simulink model "pendubotSim"  (R2016a)
settings: Solver=VariableStepAuto  StartTime=0.0  StopTime=10.0  RelTol=1e-3
InitFcn:
  | initFcn
values from neighbouring files (symbols this model uses):
  g = 9.81    [getParams.m]    (also in sFunModell.m = block.DialogPrm(1).Data)
  l1 = 0.2    [getParams.m]    (also in sFunModell.m = block.DialogPrm(4).Data)
  l2 = 0.2    [getParams.m]    (also in sFunModell.m = block.DialogPrm(5).Data)
  m1 = 0.3    [getParams.m]    (also in sFunModell.m = block.DialogPrm(2).Data)
  m2 = 0.3    [getParams.m]    (also in sFunModell.m = block.DialogPrm(3).Data)
  RP1 = 1e-2    (= 0.01)    [getParams.m]    (also in sFunModell.m = block.DialogPrm(6).Data)
  RP2 = 1e-3    (= 0.001)    [getParams.m]    (also in sFunModell.m = block.DialogPrm(7).Data)
settings Model: Creator=bened  LastModifiedBy=bened
settings GRTTargetCC: GeneratePreprocessorConditionals=Use local settings

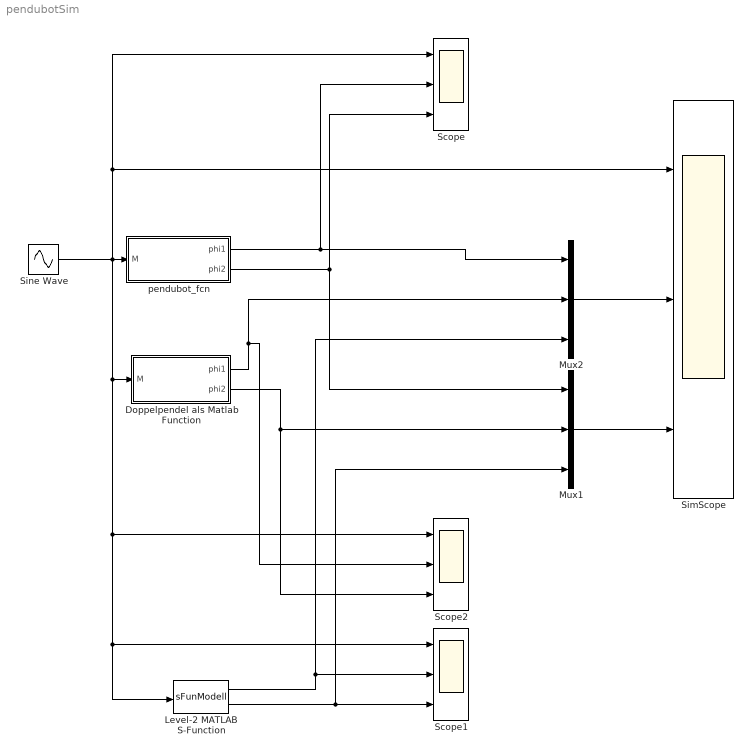
== system pendubotSim ==
  Doppelpendel als Matlab Function : Subsystem
  Level-2 MATLAB S-Function : M-S-Function  FunctionName=sFunModell  Parameters=g, m1, m2, l1, l2, RP1, RP2
  Mux1 : Mux  Inputs=3
  Mux2 : Mux  Inputs=3
  Scope : Scope  NumInputPorts=3
  Scope1 : Scope  NumInputPorts=3
  Scope2 : Scope  NumInputPorts=3
  "SimScope " : Scope  NumInputPorts=3
  Sine Wave : Sin  Amplitude=.1  SampleTime=0
  pendubot_fcn : Subsystem
  wires:
  pendubot_fcn/1(phi1) -> Mux2/1, Scope/2
  pendubot_fcn/2(phi2) -> Mux1/1, Scope/3
  Level-2 MATLAB S-Function/1 -> Mux2/3, Scope1/2
  Level-2 MATLAB S-Function/2 -> Scope1/3, Mux1/3
  Mux2/1 -> "SimScope "/2
  Mux1/1 -> "SimScope "/3
  Doppelpendel als Matlab Function/1(phi1) -> Scope2/2, Mux2/2
  Doppelpendel als Matlab Function/2(phi2) -> Scope2/3, Mux1/2
  Sine Wave/1 -> Doppelpendel als Matlab Function/1(M), Scope2/1, Level-2 MATLAB S-Function/1, Scope1/1, "SimScope "/1, Scope/1, pendubot_fcn/1(M)

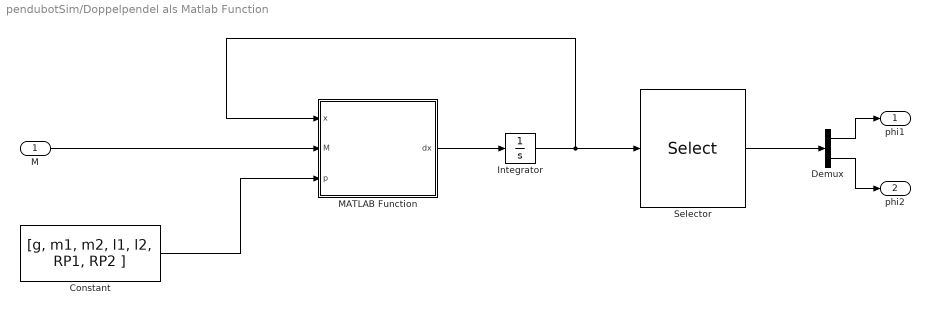
== system pendubotSim/Doppelpendel als Matlab Function ==
  M : Inport
  Constant : Constant  Value=[g, m1, m2, l1, l2, RP1, RP2 ]
  Demux : Demux  Outputs=2
  Integrator : Integrator  InitialCondition=[0 0 0 0]
  MATLAB Function : MATLAB Function  TreatAsAtomicUnit=on
  Selector : Selector  InputPortWidth=4  IndexOptions=Index vector (dialog)  Indices=[1 3]  OutputSizes=1
  phi1 : Outport
  phi2 : Outport  Port=2
  wires:
  M/1 -> MATLAB Function/2(M)
  Constant/1 -> MATLAB Function/3(p)
  MATLAB Function/1(dx) -> Integrator/1
  Integrator/1 -> Selector/1, MATLAB Function/1(x)
  Demux/1 -> phi1/1
  Demux/2 -> phi2/1
  Selector/1 -> Demux/1

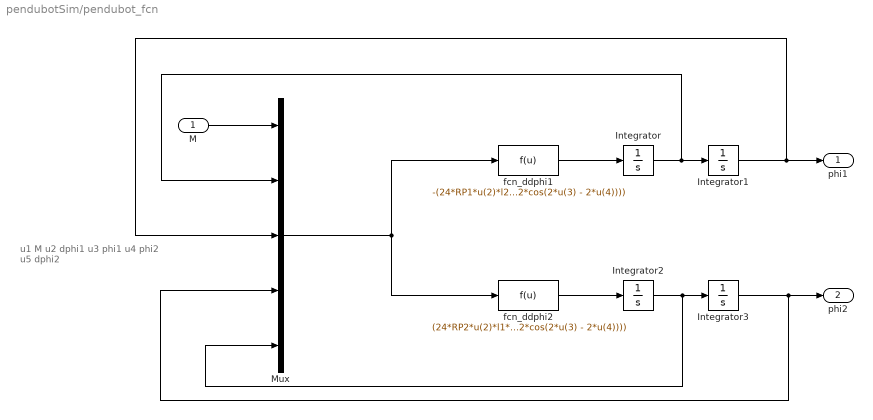
== system pendubotSim/pendubot_fcn ==
  note: u1 M
      | u2 dphi1
      | u3 phi1
      | u4 phi2
      | u5 dphi2
  M : Inport
  Integrator{,1..3} (4 alike) : Integrator
  Mux : Mux  Inputs=5
  fcn_ddphi1 : Fcn  Expr=-(24*RP1*u(2)*l2 - 24*u(1)*l2 + 36*RP2*u(2)*l1*cos(u(3) - u(4)) - 36*RP2*u(5)*l1*cos(u(3) - u(4)) + 9*g*l1*l2*m2*sin(u(3) - 2*u(4)) + 9*u(2)^2*l1^2*l2*m2*sin(2*u(3) - 2*u(4)) + 12*u(5)^2*l1*l2^2*m2*sin(u(3) - u(4)) + 12*g*l1*l2*m1*sin(u(3)) + 15*g*l1*l2*m2*sin(u(3)))/(l1^2*l2*(8*m1 + 15*m2 - 9*m2*cos(2*u(3) - 2*u(4))))
  fcn_ddphi2 : Fcn  Expr=(24*RP2*u(2)*l1*m1 - 36*u(1)*l2*m2*cos(u(3) - u(4)) + 72*RP2*u(2)*l1*m2 - 24*RP2*u(5)*l1*m1 - 72*RP2*u(5)*l1*m2 + 36*u(2)^2*l1^2*l2*m2^2*sin(u(3) - u(4)) - 18*g*l1*l2*m2^2*sin(u(4)) + 9*u(5)^2*l1*l2^2*m2^2*sin(2*u(3) - 2*u(4)) + 18*g*l1*l2*m2^2*sin(2*u(3) - u(4)) + 36*RP1*u(2)*l2*m2*cos(u(3) - u(4)) + 12*u(2)^2*l1^2*l2*m1*m2*sin(u(3) - u(4)) - 3*g*l1*l2*m1*m2*sin(u(4)) + 9*g*l1*l2*m1*m2*sin(2*u(3) - u(4)))/(l1*l2^2*m2*(8*m1 + 15*m2 - 9*m2*cos(2*u(3) - 2*u(4))))
  phi1 : Outport
  phi2 : Outport  Port=2
  wires:
  M/1 -> Mux/1
  Mux/1 -> fcn_ddphi2/1, fcn_ddphi1/1
  fcn_ddphi1/1 -> Integrator/1
  Integrator/1 -> Mux/2, Integrator1/1
  fcn_ddphi2/1 -> Integrator2/1
  Integrator2/1 -> Mux/5, Integrator3/1
  Integrator3/1 -> Mux/4, phi2/1
  Integrator1/1 -> Mux/3, phi1/1

== matlab function pendubotSim/Doppelpendel als Matlab Function/MATLAB Function ==
  data: x input; dx output; M input; p input
function dx = fcn(x,M,p)
%#codegen

phi1 = x(1);
dphi1 = x(2);
phi2 = x(3);
dphi2 = x(4);

g = p(1);
m1 = p(2);
m2 = p(3);
l1 = p(4);
l2 = p(5);
Rp1 = p(6);
Rp2 = p(7);

ddphi1 = -(24*Rp1*dphi1*l2 - 24*M*l2 + 36*Rp2*dphi1*l1*cos(phi1 - phi2) - 36*Rp2*dphi2*l1*cos(phi1 - phi2) + 9*g*l1*l2*m2*sin(phi1 - 2*phi2) + 9*dphi1^2*l1^2*l2*m2*sin(2*phi1 - 2*phi2) + 12*dphi2^2*l1*l2^2*m2*sin(phi1 - phi2) + 12*g*l1*l2*m1*sin(phi1) + 15*g*l1*l2*m2*sin(phi1))/(l1^2*l2*(8*m1 + 15*m2 - 9*m2*cos(2*phi1 - 2*phi2)));

ddphi2 = (6*(4*Rp2*dphi1*l1*m1 - 6*M*l2*m2*cos(phi1 - phi2) + 12*Rp2*dphi1*l1*m2 - 4*Rp2*dphi2*l1*m1 - 12*Rp2*dphi2*l1*m2 + 6*dphi1^2*l1^2*l2*m2^2*sin(phi1 - phi2) - 3*g*l1*l2*m2^2*sin(phi2) + (3*dphi2^2*l1*l2^2*m2^2*sin(2*phi1 - 2*phi2))/2 + 3*g*l1*l2*m2^2*sin(2*phi1 - phi2) + 6*Rp1*dphi1*l2*m2*cos(phi1 - phi2) + 2*dphi1^2*l1^2*l2*m1*m2*sin(phi1 - phi2) - (g*l1*l2*m1*m2*sin(phi2))/2 + (3*g*l1*l2*m1*m2*sin(2*phi1 - phi2))/2))/(l1*l2^2*m2*(8*m1 + 15*m2 - 9*m2*cos(2*phi1 - 2*phi2)));


dx = [dphi1, ddphi1, dphi2, ddphi2];
